simulink model "simulacao_manipulador_scara"  (R2024a)
settings: Solver=VariableStepAuto  StartTime=0.0  StopTime=10.0  RelTol=1e-3
undefined symbols (not defined in the file or in its folder): dqi, Kd, Kp, qf, qi
settings Model: Creator=alefp  LastModifiedBy=rodrigo
settings RTWCC: GPUComputeCapability=3.5

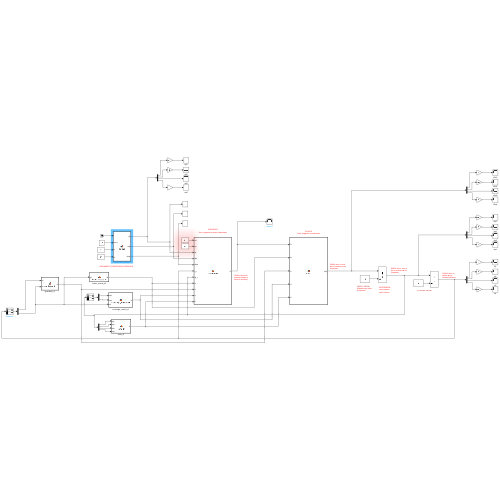
[thumbnail: Simulink's stored preview of the top-level diagram]
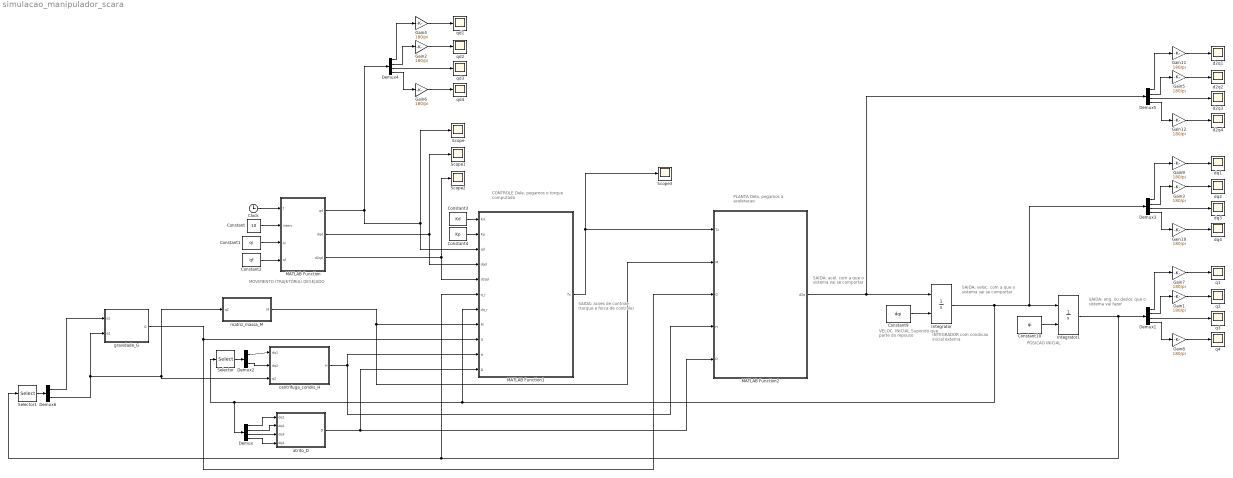
== system simulacao_manipulador_scara ==
  note: MOVIMENTO (TRAJETÓRIA) DESEJADO
  note: CONTROLE
      | Dele, pegamos o torque computado
  note: PLANTA
      | Dela, pegamos a aceleracao
  note: INTEGRADOR
      | com condicao inicial externa
  note: VELOC. INICIAL
      | Supondo que parte do repouso
  note: POSICAO INICIAL
  note: SAIDA: ang. ou desloc que o sistema vai fazer
  note: SAIDA: veloc. com a que o sistema vai se comportar
  note: SAIDA: acel. com a que o sistema vai se comportar
  note: SAIDA: acoes de controle (torque e forca de controle)
  Clock : Clock
  Constant : Constant  Value=10
  Constant1 : Constant  Value=qi
  Constant10 : Constant  Value=qi
  Constant2 : Constant  Value=qf
  Constant3 : Constant  Value=Kd
  Constant4 : Constant  Value=Kp
  Constant9 : Constant  Value=dqi
  Demux{,1,3..5} (5 alike) : Demux
  Demux2 : Demux  Outputs=2
  Demux6 : Demux  Outputs=2
  Gain{1..12} (12 alike) : Gain  Gain=180/pi
  Integrator : Integrator  InitialConditionSource=external
  Integrator1 : Integrator  InitialConditionSource=external
  MATLAB Function : MATLAB Function  TreatAsAtomicUnit=on
  MATLAB Function1 : MATLAB Function  TreatAsAtomicUnit=on
  MATLAB Function2 : MATLAB Function  TreatAsAtomicUnit=on
  Scope{,1..3} (4 alike) : Scope
  Selector : Selector  InputPortWidth=4  IndexOptions=Index vector (dialog)  Indices=[1, 2]  OutputSizes=1
  Selector1 : Selector  InputPortWidth=4  IndexOptions=Index vector (dialog)  Indices=[1, 2]  OutputSizes=1
  atrito_D : MATLAB Function  TreatAsAtomicUnit=on
  centrifuga_coriolis_H : MATLAB Function  TreatAsAtomicUnit=on
  d2q{1..4} (4 alike) : Scope
  dq{1..4} (4 alike) : Scope
  gravidade_G : MATLAB Function  TreatAsAtomicUnit=on
  matriz_massa_M : MATLAB Function  TreatAsAtomicUnit=on
  q{1..4} (4 alike) : Scope
  qd{1..4} (4 alike) : Scope
  wires:
  MATLAB Function/2(dqd) -> MATLAB Function1/4(dqd), Scope1/1
  MATLAB Function/3(d2qd) -> MATLAB Function1/5(d2qd), Scope2/1
  MATLAB Function/1(qd) -> Scope/1, MATLAB Function1/3(qd), Demux4/1
  Constant/1 -> MATLAB Function/2(interv)
  Constant1/1 -> MATLAB Function/3(qi)
  Clock/1 -> MATLAB Function/1(t)
  Constant2/1 -> MATLAB Function/4(qf)
  MATLAB Function1/1(Tc) -> Scope3/1, MATLAB Function2/1(Tc)
  Constant9/1 -> Integrator/2
  Constant10/1 -> Integrator1/2
  Demux4/1 -> Gain4/1
  Gain4/1 -> qd1/1
  Demux4/3 -> qd3/1
  matriz_massa_M/1(M) -> MATLAB Function2/2(M), MATLAB Function1/8(M)
  gravidade_G/1(G) -> MATLAB Function1/9(G), MATLAB Function2/3(G)
  centrifuga_coriolis_H/1(H) -> MATLAB Function1/10(H), MATLAB Function2/4(H)
  atrito_D/1(D) -> MATLAB Function1/11(D), MATLAB Function2/5(D)
  Gain2/1 -> qd2/1
  Demux4/2 -> Gain2/1
  Gain6/1 -> qd4/1
  Demux4/4 -> Gain6/1
  Demux/1 -> atrito_D/1(dq1)
  Demux/2 -> atrito_D/2(dq2)
  Demux/3 -> atrito_D/3(dq3)
  Demux/4 -> atrito_D/4(dq4)
  Demux2/2 -> centrifuga_coriolis_H/2(dq2)
  Demux2/1 -> centrifuga_coriolis_H/1(dq1)
  Selector/1 -> Demux2/1
  Demux6/2 -> gravidade_G/2(q2), matriz_massa_M/1(q2), centrifuga_coriolis_H/3(q2)
  Demux6/1 -> gravidade_G/1(q1)
  Selector1/1 -> Demux6/1
  Demux1/4 -> Gain8/1
  Demux1/3 -> q3/1
  Demux1/1 -> Gain7/1
  Demux1/2 -> Gain1/1
  Integrator1/1 -> MATLAB Function1/6(q_r), Selector1/1, Demux1/1
  Gain1/1 -> q2/1
  Gain8/1 -> q4/1
  Gain7/1 -> q1/1
  Demux3/4 -> Gain10/1
  Demux3/3 -> dq3/1
  Demux3/1 -> Gain9/1
  Demux3/2 -> Gain3/1
  Integrator/1 -> Demux3/1, Integrator1/1, Selector/1, Demux/1, MATLAB Function1/7(dq_r)
  Gain3/1 -> dq2/1
  Gain10/1 -> dq4/1
  Gain9/1 -> dq1/1
  Demux5/4 -> Gain12/1
  Demux5/3 -> d2q3/1
  Demux5/1 -> Gain11/1
  Demux5/2 -> Gain5/1
  MATLAB Function2/1(d2q) -> Demux5/1, Integrator/1
  Gain5/1 -> d2q2/1
  Gain12/1 -> d2q4/1
  Gain11/1 -> d2q1/1
  Constant3/1 -> MATLAB Function1/1(Kd)
  Constant4/1 -> MATLAB Function1/2(Kp)

== matlab function simulacao_manipulador_scara/MATLAB Function1 ==
  data: Kd input; Kp input; Tc output; qd input; dqd input; d2qd input; q_r input; dq_r input; M input; G input; H input; D input
function Tc  = controlador(Kd, Kp, qd, dqd, d2qd, q_r, dq_r, M, G, H, D)
Tc = M*(d2qd + Kd*(dqd-dq_r) + Kp*(qd- q_r)) + H + G + D;

== matlab function simulacao_manipulador_scara/MATLAB Function ==
  data: t input; qd output; interv input; qi input; qf input; dqd output; d2qd output
function [qd, dqd, d2qd] = cinCub(t, interv, qi, qf)

tf = interv;
A = [1 0 0 0; 0 1 0 0; 1 tf tf^2 tf^3; 0 1 2*tf 3*tf^2]
b = [qi(1); 0; qf(1); 0];
x = inv(A)*b;

qd = zeros(4,1);
dqd = qd;
d2qd = qd;


qd(1,1) = x(1) + x(2)*t + x(3)*t^2 + x(4)*t^3;
dqd(1,1) = x(2) + 2*x(3)*t + 3*x(4)*t^2;
d2qd(1,1) = 2*x(3) + 6*x(4)*t;


b = [qi(2); 0; qf(2); 0];
x = inv(A)*b;

qd(2,1) = x(1) + x(2)*t + x(3)*t^2 + x(4)*t^3;
dqd(2,1) = x(2) + 2*x(3)*t + 3*x(4)*t^2;
d2qd(2,1) = 2*x(3) + 6*x(4)*t;


b = [qi(3); 0; qf(3); 0];
x = inv(A)*b;

qd(3,1) = x(1) + x(2)*t + x(3)*t^2 + x(4)*t^3;
dqd(3,1) = x(2) + 2*x(3)*t + 3*x(4)*t^2;
d2qd(3,1) = 2*x(3) + 6*x(4)*t;

b = [qi(4); 0; qf(4); 0];
x = inv(A)*b;

qd(4,1) = x(1) + x(2)*t + x(3)*t^2 + x(4)*t^3;
dqd(4,1) = x(2) + 2*x(3)*t + 3*x(4)*t^2;
d2qd(4,1) = 2*x(3) + 6*x(4)*t;

== matlab function simulacao_manipulador_scara/MATLAB Function2 ==
  data: d2q output; Tc input; M input; G input; H input; D input
function d2q  = planta(Tc, M, G, H, D) % a planta devolve a aceleração simulada
d2q = M\(Tc-H-G-D);

== matlab function simulacao_manipulador_scara/matriz_massa_M ==
  data: q2 input; M output
function M = matriz_massa_M(q2)
%#codegen

%    This function was generated by the Symbolic Math Toolbox version 24.1.
%    08-Sep-2024 19:28:31

% q2 = complex(q2);  % if required to enforce complex operations
t2 = cos(q2);
t3 = t2.*(1.17e+2./2.0e+2);
t4 = t3+6.3e+1./2.5e+2;
M = reshape([t2.*(1.17e+2./1.0e+2)+1.911375,t4,0.0,0.0,t4,3.908708333333333e-1,1.155375e-1,3.96e-2,0.0,1.155375e-1,1.3155375,3.96e-2,0.0,3.96e-2,3.96e-2,3.96e-2],[4,4]);
end

== matlab function simulacao_manipulador_scara/gravidade_G ==
  data: q1 input; G output; q2 input
function G = gravidade_G(q1,q2)
%#codegen

%    This function was generated by the Symbolic Math Toolbox version 24.1.
%    08-Sep-2024 19:28:31

% q1 = complex(q1);  % if required to enforce complex operations
% q2 = complex(q2);  % if required to enforce complex operations
t2 = q1+q2;
t3 = cos(t2);
t4 = t3.*7.6518;
t5 = -t4;
G = [t5-cos(q1).*2.3544e+1;t5;0.0;0.0];
end

== matlab function simulacao_manipulador_scara/centrifuga_coriolis_H ==
  data: dq1 input; H output; dq2 input; q2 input
function H = centrifuga_coriolis_H(dq1,dq2,q2)
%#codegen

%    This function was generated by the Symbolic Math Toolbox version 24.1.
%    08-Sep-2024 19:28:31

% dq1 = complex(dq1);  % if required to enforce complex operations
% dq2 = complex(dq2);  % if required to enforce complex operations
% q2 = complex(q2);  % if required to enforce complex operations
t2 = sin(q2);
H = [dq2.*t2.*(dq1.*2.0+dq2).*(-1.17e+2./2.0e+2);dq1.^2.*t2.*(1.17e+2./2.0e+2);0.0;0.0];
end

== matlab function simulacao_manipulador_scara/atrito_D ==
  data: dq1 input; D output; dq2 input; dq3 input; dq4 input
function D = atrito_D(dq1,dq2,dq3,dq4)
%#codegen

%    This function was generated by the Symbolic Math Toolbox version 24.1.
%    08-Sep-2024 19:28:32

% dq1 = complex(dq1);  % if required to enforce complex operations
% dq2 = complex(dq2);  % if required to enforce complex operations
% dq3 = complex(dq3);  % if required to enforce complex operations
% dq4 = complex(dq4);  % if required to enforce complex operations
D = [dq1./1.0e+2;dq2./1.0e+2;dq3.*(3.0./4.0e+2);dq4.*(3.0./2.5e+2)];
end
